simulink model "ADPLL_base"  (R2017a)
settings: Solver=ode23  StartTime=0.0  StopTime=4e-4  RelTol=1e-3
values from neighbouring files (symbols this model uses):
  Ki = 0.01    [ADPLL_script_autocor.m]    (also in ADPLL_script_base.m; ADPLL_script_nn.m)
  Kp = Kp_int/(Kp_max+1)    (= 0.0390625)    [ADPLL_script_autocor.m]    (also in ADPLL_script_base.m = 0.1; ADPLL_script_nn.m)
  N = 10    [ADPLL_script_autocor.m]    (also in ADPLL_script_base.m; ADPLL_script_nn.m)
undefined symbols (not defined in the file or in its folder): BBPFD_delay, DCO_Noise, DCO_Seed, Ffree, Fref, Kdco, Ref_Noise, Ref_Seed
libraries: simulink_extras x3, simulink x2
settings Model: Creator=ECL328  LastModifiedBy=frans

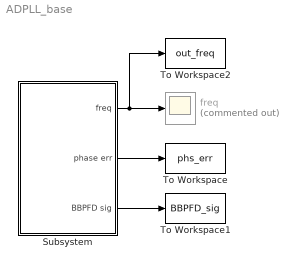
== system ADPLL_base ==
  Subsystem : Subsystem  mask{N=N, Kp=Kp, Ki=Ki, Kdco=Kdco, Fref=Fref, Ffree=Ffree, BBPFD_delay=BBPFD_delay, DCO_Noise=DCO_Noise, Ref_Noise=Ref_Noise}
  To Workspace : ToWorkspace  VariableName=phs_err  SampleTime=-1
  To Workspace1 : ToWorkspace  VariableName=BBPFD_sig  SampleTime=-1
  To Workspace2 : ToWorkspace  VariableName=out_freq  SampleTime=-1
  freq : Scope  Commented=on
  wires:
  Subsystem/1(freq) -> To Workspace2/1, freq/1
  Subsystem/2(phase err) -> To Workspace/1
  Subsystem/3(BBPFD sig) -> To Workspace1/1

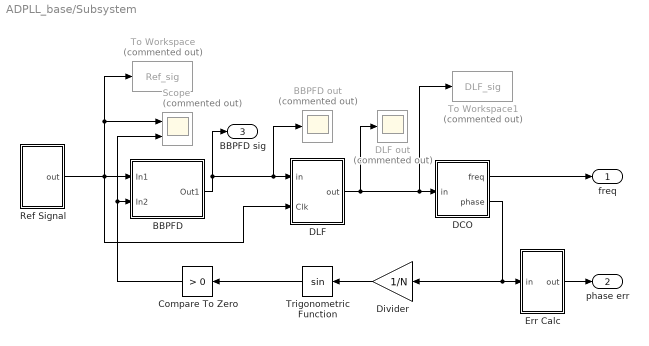
== system ADPLL_base/Subsystem ==
  BBPFD : Subsystem
  BBPFD out : Scope  Commented=on
  Compare To Zero : simulink/Logic and Bit Operations/Compare To Zero  relop=>  OutDataTypeStr=boolean
  DCO : Subsystem
  DLF : Subsystem
  DLF out : Scope  Commented=on
  Divider : Gain  Gain=1/N
  Err Calc : Subsystem
  Ref Signal : Subsystem
  Scope : Scope  Commented=on  NumInputPorts=2
  To Workspace : ToWorkspace  Commented=on  VariableName=Ref_sig  SampleTime=-1
  To Workspace1 : ToWorkspace  Commented=on  VariableName=DLF_sig  SampleTime=-1
  Trigonometric Function : Trigonometry
  freq : Outport
  phase err : Outport  Port=2
  BBPFD sig : Outport  Port=3
  wires:
  BBPFD/1(Out1) -> BBPFD out/1, DLF/1(in), BBPFD sig/1
  Divider/1 -> Trigonometric Function/1
  DLF/1(out) -> DLF out/1, To Workspace1/1, DCO/1(in)
  DCO/1(freq) -> freq/1
  Err Calc/1(out) -> phase err/1
  Trigonometric Function/1 -> Compare To Zero/1
  Compare To Zero/1 -> Scope/2, BBPFD/2(In2)
  Ref Signal/1(out) -> To Workspace/1, Scope/1, DLF/2(Clk), BBPFD/1(In1)
  DCO/2(phase) -> Err Calc/1(in), Divider/1

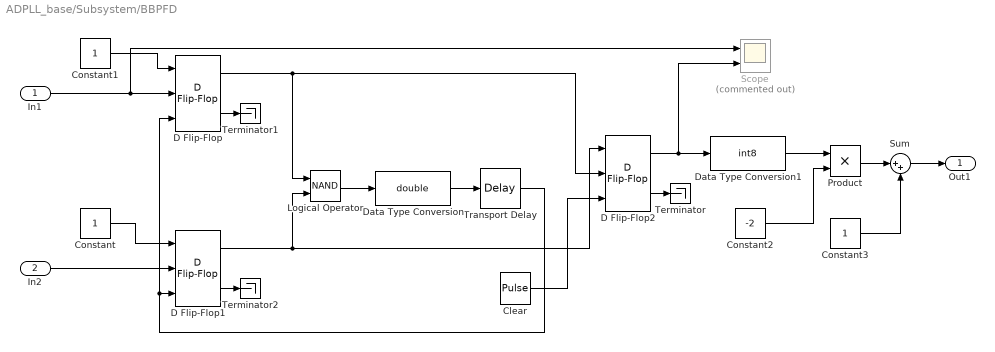
== system ADPLL_base/Subsystem/BBPFD ==
  In1 : Inport
  In2 : Inport  Port=2
  Clear : DiscretePulseGenerator  PulseType=Time based  Period=20  PulseWidth=50
  Constant : Constant  OutDataTypeStr=boolean
  Constant1 : Constant  OutDataTypeStr=boolean
  Constant2 : Constant  Value=-2
  Constant3 : Constant
  D Flip-Flop : simulink_extras/Flip Flops/D Flip-Flop
      settings: SourceProductName=Simulink
  D Flip-Flop1 : simulink_extras/Flip Flops/D Flip-Flop
      settings: SourceProductName=Simulink
  D Flip-Flop2 : simulink_extras/Flip Flops/D Flip-Flop
      settings: SourceProductName=Simulink
  Data Type Conversion : DataTypeConversion  OutDataTypeStr=double
  Data Type Conversion1 : DataTypeConversion  OutDataTypeStr=int8
  Logical Operator : Logic  Operator=NAND  AllPortsSameDT=off  OutDataTypeStr=boolean
  Product : Product
  Scope : Scope  Commented=on  NumInputPorts=2
  Sum : Sum  Inputs=|++
  Terminator : Terminator
  Terminator1 : Terminator
  Terminator2 : Terminator
  Transport Delay : TransportDelay  DelayTime=BBPFD_delay
  Out1 : Outport
  wires:
  Data Type Conversion/1 -> Transport Delay/1
  Constant/1 -> D Flip-Flop1/1
  Sum/1 -> Out1/1
  D Flip-Flop2/1 -> Scope/2, Data Type Conversion1/1
  Product/1 -> Sum/1
  In1/1 -> Scope/1, D Flip-Flop/2
  Clear/1 -> D Flip-Flop2/3
  D Flip-Flop2/2 -> Terminator/1
  In2/1 -> D Flip-Flop1/2
  Constant3/1 -> Sum/2
  Data Type Conversion1/1 -> Product/1
  Constant1/1 -> D Flip-Flop/1
  Transport Delay/1 -> D Flip-Flop/3, D Flip-Flop1/3
  D Flip-Flop/1 -> D Flip-Flop2/2, Logical Operator/1
  D Flip-Flop1/1 -> D Flip-Flop2/1, Logical Operator/2
  Logical Operator/1 -> Data Type Conversion/1
  D Flip-Flop1/2 -> Terminator2/1
  Constant2/1 -> Product/2
  D Flip-Flop/2 -> Terminator1/1

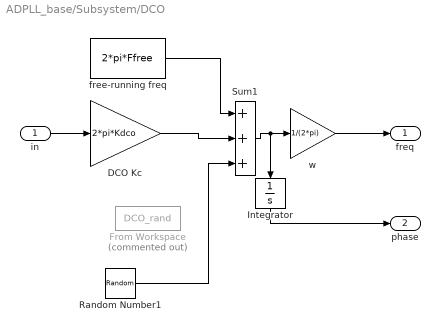
== system ADPLL_base/Subsystem/DCO ==
  in : Inport
  DCO Kc : Gain  Gain=2*pi*Kdco
  From Workspace : FromWorkspace  Commented=on  VariableName=DCO_rand  SampleTime=0
  Integrator : Integrator  WrapState=on  WrappedStateUpperValue=2*N*pi  WrappedStateLowerValue=0
  Random Number1 : RandomNumber  Variance=DCO_Noise  Seed=DCO_Seed  SampleTime=1/(Fref*4)
  Sum1 : Sum  Inputs=+++
  free-running freq : Constant  Value=2*pi*Ffree
  w : Gain  Gain=1/(2*pi)
  freq : Outport
  phase : Outport  Port=2
  wires:
  in/1 -> DCO Kc/1
  Integrator/1 -> phase/1
  DCO Kc/1 -> Sum1/2
  Sum1/1 -> w/1, Integrator/1
  free-running freq/1 -> Sum1/1
  w/1 -> freq/1
  Random Number1/1 -> Sum1/3

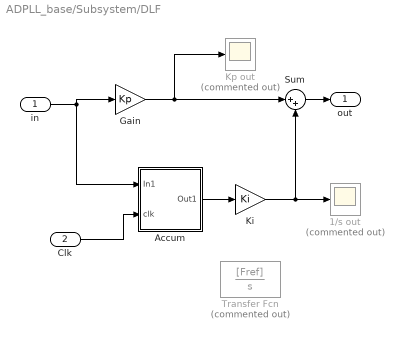
== system ADPLL_base/Subsystem/DLF ==
  in : Inport
  Clk : Inport  Port=2
  1/s out : Scope  Commented=on
  Accum : Subsystem
  Gain : Gain  Gain=Kp
  Ki : Gain  Gain=Ki
  Kp out : Scope  Commented=on
  Sum : Sum  Inputs=|++
  Transfer Fcn : TransferFcn  Commented=on  Numerator=[Fref]  Denominator=[1 0]
  out : Outport
  wires:
  Accum/1(Out1) -> Ki/1
  Gain/1 -> Kp out/1, Sum/1
  Sum/1 -> out/1
  in/1 -> Gain/1, Accum/1(In1)
  Clk/1 -> Accum/2(clk)
  Ki/1 -> Sum/2, 1/s out/1

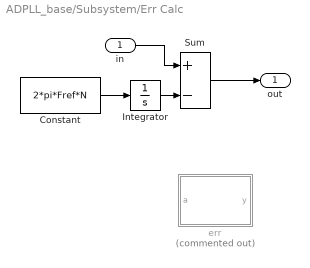
== system ADPLL_base/Subsystem/Err Calc ==
  in : Inport
  Constant : Constant  Value=2*pi*Fref*N
  Integrator : Integrator  WrapState=on  WrappedStateUpperValue=2*N*pi  WrappedStateLowerValue=0
  Sum : Sum  Inputs=+-
  err : MATLAB Function  Commented=on  TreatAsAtomicUnit=on
  out : Outport
  wires:
  Constant/1 -> Integrator/1
  Integrator/1 -> Sum/2
  in/1 -> Sum/1
  Sum/1 -> out/1

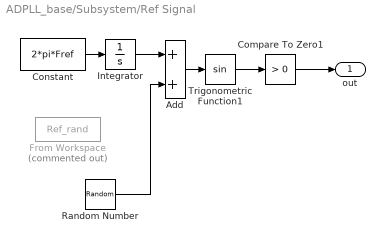
== system ADPLL_base/Subsystem/Ref Signal ==
  Add : Sum
  Compare To Zero1 : simulink/Logic and Bit Operations/Compare To Zero  relop=>  OutDataTypeStr=boolean
  Constant : Constant  Value=2*pi*Fref
  From Workspace : FromWorkspace  Commented=on  VariableName=Ref_rand  SampleTime=0
  Integrator : Integrator  WrapState=on  WrappedStateUpperValue=2*pi  WrappedStateLowerValue=0
  Random Number : RandomNumber  Variance=Ref_Noise  Seed=Ref_Seed  SampleTime=1/(4*Fref)
  Trigonometric Function1 : Trigonometry
  out : Outport
  wires:
  Integrator/1 -> Add/1
  Constant/1 -> Integrator/1
  Add/1 -> Trigonometric Function1/1
  Trigonometric Function1/1 -> Compare To Zero1/1
  Compare To Zero1/1 -> out/1
  Random Number/1 -> Add/2

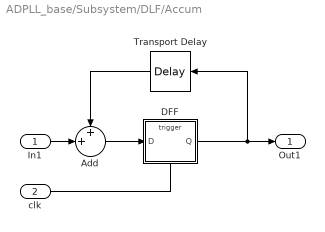
== system ADPLL_base/Subsystem/DLF/Accum ==
  In1 : Inport
  clk : Inport  Port=2
  Add : Sum  Inputs=++|
  DFF : Subsystem
  Transport Delay : TransportDelay  DelayTime=BBPFD_delay
  Out1 : Outport
  wires:
  In1/1 -> Add/2
  DFF/1(Q) -> Transport Delay/1, Out1/1
  Transport Delay/1 -> Add/1
  clk/1 -> DFF/Trigger
  Add/1 -> DFF/1(D)

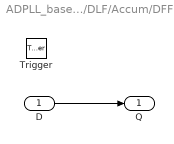
== system ADPLL_base/Subsystem/DLF/Accum/DFF ==
  D : Inport
  Trigger : TriggerPort  VariantControl=Variant  PortDimensions=1
  Q : Outport
  wires:
  D/1 -> Q/1

== matlab function ADPLL_base/Subsystem/Err Calc/err ==
  data: a input; y output
function y = fcn(a)
temp = rem(a,2*pi);
y = temp - (2*pi)*(temp>pi);
